simulink model "Static_Controller_With_Observer"  (R2019a)
settings: Solver=VariableStepAuto  StartTime=0.0  StopTime=50  RelTol=1e-3
values from neighbouring files (symbols this model uses):
  K = K(1:3)    [ask4.m]
  L = acker(A',C',5*[p1 p2 p3 ])'    [ask4.m]
undefined symbols (not defined in the file or in its folder): A, B, C, N
settings Model: Creator=kyria  LastModifiedBy=kyria

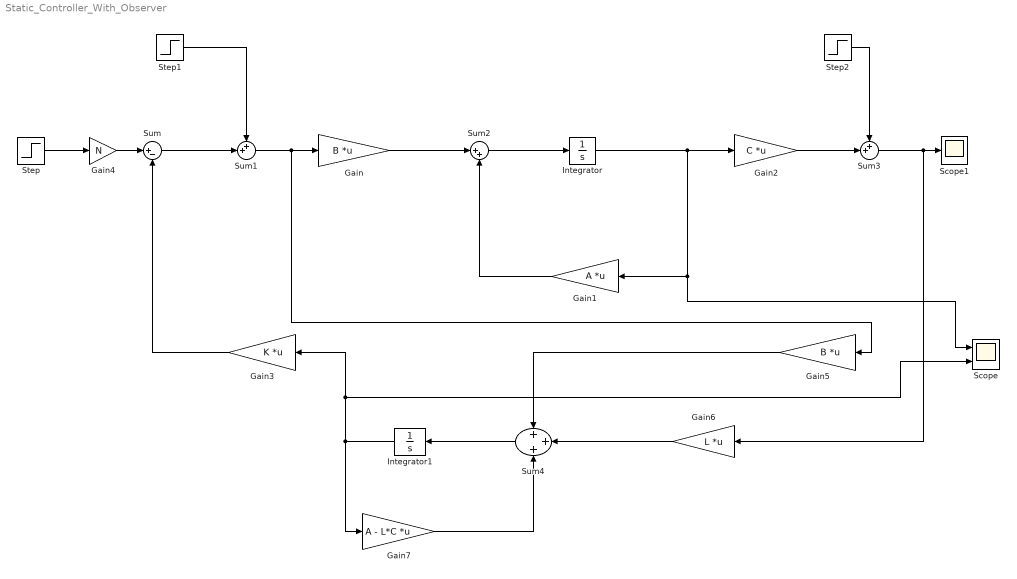
== system Static_Controller_With_Observer ==
  Gain : Gain  Gain=B  Multiplication=Matrix(K*u)
  Gain1 : Gain  Gain=A  Multiplication=Matrix(K*u)
  Gain2 : Gain  Gain=C  Multiplication=Matrix(K*u)
  Gain3 : Gain  Gain=K  Multiplication=Matrix(K*u)
  Gain4 : Gain  Gain=N
  Gain5 : Gain  Gain=B  Multiplication=Matrix(K*u)
  Gain6 : Gain  Gain=L  Multiplication=Matrix(K*u)
  Gain7 : Gain  Gain=A - L*C  Multiplication=Matrix(K*u)
  Integrator : Integrator
  Integrator1 : Integrator
  Scope : Scope  NumInputPorts=2
  Scope1 : Scope
  Step : Step  Time=0  Before=1  SampleTime=0
  Step1 : Step  Time=30  SampleTime=0
  Step2 : Step  Time=15  SampleTime=0
  Sum : Sum  Inputs=|+-
  Sum1 : Sum  Inputs=++|
  Sum2 : Sum  Inputs=|++
  Sum3 : Sum  Inputs=++|
  Sum4 : Sum  Inputs=+++
  wires:
  Step/1 -> Gain4/1
  Sum/1 -> Sum1/2
  Step1/1 -> Sum1/1
  Sum1/1 -> Gain5/1, Gain/1
  Gain/1 -> Sum2/1
  Sum2/1 -> Integrator/1
  Gain1/1 -> Sum2/2
  Integrator/1 -> Scope/1, Gain1/1, Gain2/1
  Gain3/1 -> Sum/2
  Gain2/1 -> Sum3/2
  Step2/1 -> Sum3/1
  Sum3/1 -> Gain6/1, Scope1/1
  Gain4/1 -> Sum/1
  Gain5/1 -> Sum4/1
  Gain6/1 -> Sum4/2
  Gain7/1 -> Sum4/3
  Sum4/1 -> Integrator1/1
  Integrator1/1 -> Gain7/1, Scope/2, Gain3/1
